simulink model "simula_axeboat"  (Simulink 8.5)
settings: Solver=ode45  StartTime=0.0  StopTime=1  MaxStep=0.01  RelTol=1e-6
values from neighbouring files (symbols this model uses):
  Ac = diag([(Ae-Bv)/M (Ae-Bvn)/M (Ae*b*b - Bw)/J])    [robo_LQR.m]
  Bc = [0 sqrt(3)/(2*M) -sqrt(3)/(2*M) ; -1/M 1/(2*M) 1/(2*M) ; b/J b/J b/J]*Be    [robo_LQR.m]
  Cc = I    [robo_LQR.m]
  deltaS = [deltaSv;deltaSvn;deltaSw]    [robo_LQR.m]
  Gc = Z    [robo_LQR.m]
  Kc = Z    [robo_LQR.m]
  ts = 0.06    [robo_LQR.m]
  Vnref = 0    [robo_LQR.m]
  Vref = 0.4    [robo_LQR.m]
  Vs = [Vsv;Vsvn;Vsw]    [robo_LQR.m]
  Wref = 0    [robo_LQR.m]
undefined symbols (not defined in the file or in its folder): Kdlqry, up
libraries: simulink x1
settings Model: Creator=tito  LastModifiedBy=Jessivaldo
settings DebuggingCC: SolverPrmCheckMsg=warning  FcnCallInpInsideContextMsg=UseLocalSettings

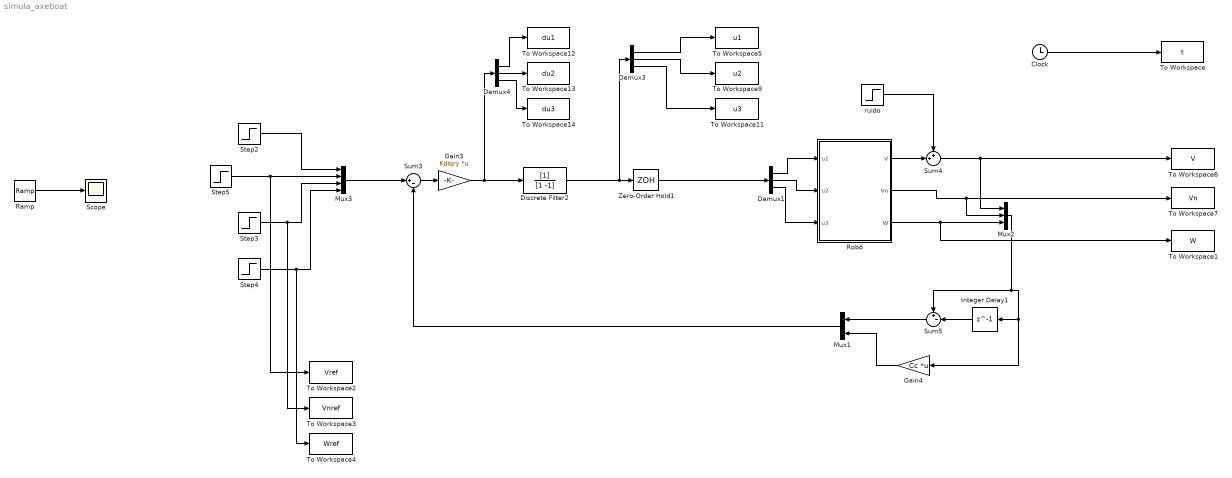
== system simula_axeboat ==
  Clock : Clock
  Demux1 : Demux  Outputs=3
  Demux3 : Demux  Outputs=3
  Demux4 : Demux  Outputs=3
  Discrete Filter2 : DiscreteFilter  Denominator=[1 -1]  SampleTime=ts
  Gain3 : Gain  Gain=Kdlqry  Multiplication=Matrix(K*u)  SampleTime=ts
  Gain4 : Gain  Gain=Cc  Multiplication=Matrix(K*u)  SampleTime=ts
  Integer Delay1 : Delay  DelayLength=1  InputProcessing=Inherited  SampleTime=ts
  Mux1 : Mux  Inputs=2
  Mux2 : Mux  Inputs=3
  Mux3 : Mux
  Ramp : simulink/Sources/Ramp  slope=0.5  start=0.5  X0=-0.6
  Robô : Subsystem
  Scope : Scope
  Step2 : Step  Time=0.1  After=[0 0 0]  SampleTime=0
  Step3 : Step  Time=0.1  After=Vnref  SampleTime=0
  Step4 : Step  Time=0.1  After=Wref  SampleTime=0
  Step5 : Step  Time=0.1  After=Vref  SampleTime=0
  Sum3 : Sum  Inputs=|+-
  Sum4 : Sum  Inputs=++|
  Sum5 : Sum  Inputs=+-|
  To Workspace : ToWorkspace  VariableName=t  SampleTime=ts
  To Workspace1 : ToWorkspace  VariableName=W  SampleTime=ts
  To Workspace11 : ToWorkspace  VariableName=u3  SampleTime=ts
  To Workspace12 : ToWorkspace  VariableName=du1  SampleTime=ts
  To Workspace13 : ToWorkspace  VariableName=du2  SampleTime=ts
  To Workspace14 : ToWorkspace  VariableName=du3  SampleTime=ts
  To Workspace2 : ToWorkspace  VariableName=Vref  SampleTime=ts
  To Workspace3 : ToWorkspace  VariableName=Vnref  SampleTime=ts
  To Workspace4 : ToWorkspace  VariableName=Wref  SampleTime=ts
  To Workspace5 : ToWorkspace  VariableName=u1  SampleTime=ts
  To Workspace6 : ToWorkspace  VariableName=V  SampleTime=ts
  To Workspace7 : ToWorkspace  VariableName=Vn  SampleTime=ts
  To Workspace9 : ToWorkspace  VariableName=u2  SampleTime=ts
  Zero-Order Hold1 : ZeroOrderHold  SampleTime=ts
  ruido : Step  Time=0.5  After=up  SampleTime=0
  wires:
  Clock/1 -> To Workspace/1
  Zero-Order Hold1/1 -> Demux1/1
  Mux2/1 -> Gain4/1, Integer Delay1/1, Sum5/1
  Discrete Filter2/1 -> Zero-Order Hold1/1, Demux3/1
  Robô/2(Vn) -> To Workspace7/1, Mux2/2
  Mux1/1 -> Sum3/2
  Sum5/1 -> Mux1/1
  Gain4/1 -> Mux1/2
  Integer Delay1/1 -> Sum5/2
  Sum3/1 -> Gain3/1
  Gain3/1 -> Discrete Filter2/1, Demux4/1
  Robô/3(W) -> To Workspace1/1, Mux2/3
  Demux3/1 -> To Workspace5/1
  Demux3/2 -> To Workspace9/1
  Demux3/3 -> To Workspace11/1
  Demux4/1 -> To Workspace12/1
  Demux4/2 -> To Workspace13/1
  Demux4/3 -> To Workspace14/1
  Demux1/1 -> Robô/1(u1)
  Demux1/2 -> Robô/2(u2)
  Demux1/3 -> Robô/3(u3)
  ruido/1 -> Sum4/1
  Robô/1(V) -> Sum4/2
  Sum4/1 -> Mux2/1, To Workspace6/1
  Mux3/1 -> Sum3/1
  Step2/1 -> Mux3/1
  Step3/1 -> To Workspace3/1, Mux3/3
  Step4/1 -> To Workspace4/1, Mux3/4
  Step5/1 -> To Workspace2/1, Mux3/2
  Ramp/1 -> Scope/1

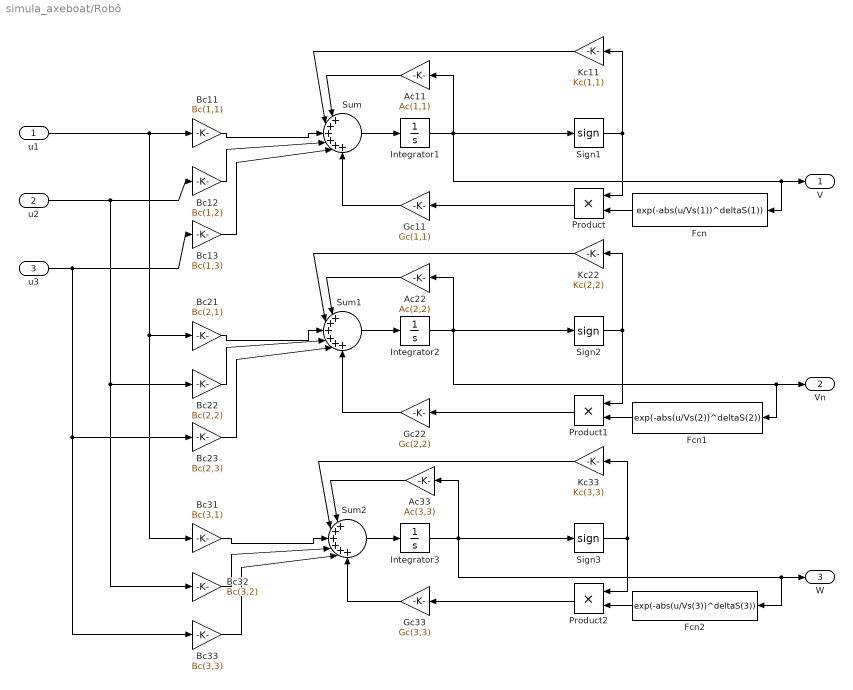
== system simula_axeboat/Robô ==
  u1 : Inport
  u2 : Inport  Port=2
  u3 : Inport  Port=3
  Ac11 : Gain  Gain=Ac(1,1)
  Ac22 : Gain  Gain=Ac(2,2)
  Ac33 : Gain  Gain=Ac(3,3)
  Bc11 : Gain  Gain=Bc(1,1)
  Bc12 : Gain  Gain=Bc(1,2)
  Bc13 : Gain  Gain=Bc(1,3)
  Bc21 : Gain  Gain=Bc(2,1)
  Bc22 : Gain  Gain=Bc(2,2)
  Bc23 : Gain  Gain=Bc(2,3)
  Bc31 : Gain  Gain=Bc(3,1)
  Bc32 : Gain  Gain=Bc(3,2)
  Bc33 : Gain  Gain=Bc(3,3)
  Fcn : Fcn  Expr=exp(-abs(u/Vs(1))^deltaS(1))
  Fcn1 : Fcn  Expr=exp(-abs(u/Vs(2))^deltaS(2))
  Fcn2 : Fcn  Expr=exp(-abs(u/Vs(3))^deltaS(3))
  Gc11 : Gain  Gain=Gc(1,1)
  Gc22 : Gain  Gain=Gc(2,2)
  Gc33 : Gain  Gain=Gc(3,3)
  Integrator1 : Integrator
  Integrator2 : Integrator
  Integrator3 : Integrator
  Kc11 : Gain  Gain=Kc(1,1)
  Kc22 : Gain  Gain=Kc(2,2)
  Kc33 : Gain  Gain=Kc(3,3)
  Product : Product  RndMeth=Zero
  Product1 : Product  RndMeth=Zero
  Product2 : Product  RndMeth=Zero
  Sign1 : Signum  ZeroCross=off
  Sign2 : Signum  ZeroCross=off
  Sign3 : Signum  ZeroCross=off
  Sum : Sum  Inputs=|++++++
  Sum1 : Sum  Inputs=|++++++
  Sum2 : Sum  Inputs=|++++++
  V : Outport
  Vn : Outport  Port=2
  W : Outport  Port=3
  wires:
  Gc33/1 -> Sum2/6
  Gc22/1 -> Sum1/6
  Gc11/1 -> Sum/6
  Fcn2/1 -> Product2/2
  Fcn1/1 -> Product1/2
  Fcn/1 -> Product/2
  Kc33/1 -> Sum2/2
  Kc22/1 -> Sum1/2
  Kc11/1 -> Sum/2
  Product2/1 -> Gc33/1
  Product1/1 -> Gc22/1
  Product/1 -> Gc11/1
  Bc33/1 -> Sum2/5
  Bc32/1 -> Sum2/4
  Bc31/1 -> Sum2/3
  Sign3/1 -> Product2/1, Kc33/1
  Ac33/1 -> Sum2/1
  Integrator3/1 -> Fcn2/1, W/1, Sign3/1, Ac33/1
  Sum2/1 -> Integrator3/1
  Bc23/1 -> Sum1/5
  Bc22/1 -> Sum1/4
  Bc21/1 -> Sum1/3
  Sign2/1 -> Product1/1, Kc22/1
  Ac22/1 -> Sum1/1
  Integrator2/1 -> Fcn1/1, Vn/1, Sign2/1, Ac22/1
  Sum1/1 -> Integrator2/1
  Bc13/1 -> Sum/5
  Bc12/1 -> Sum/4
  Bc11/1 -> Sum/3
  Sign1/1 -> Product/1, Kc11/1
  Ac11/1 -> Sum/1
  Integrator1/1 -> Fcn/1, V/1, Sign1/1, Ac11/1
  Sum/1 -> Integrator1/1
  u3/1 -> Bc33/1, Bc23/1, Bc13/1
  u2/1 -> Bc32/1, Bc22/1, Bc12/1
  u1/1 -> Bc31/1, Bc21/1, Bc11/1
